simulink model "Regulateur_Proportionel_Integrale"  (R2017a)
settings: Solver=VariableStepAuto  StartTime=0.0  StopTime=20  RelTol=1e-3
values from neighbouring files (symbols this model uses):
  Ti1 = 0.01    [declaration_des_variables.m]
  Ti2 = 0.1    [declaration_des_variables.m]
  Ti3 = 1    [declaration_des_variables.m]
settings Model: Creator=PC  LastModifiedBy=PC

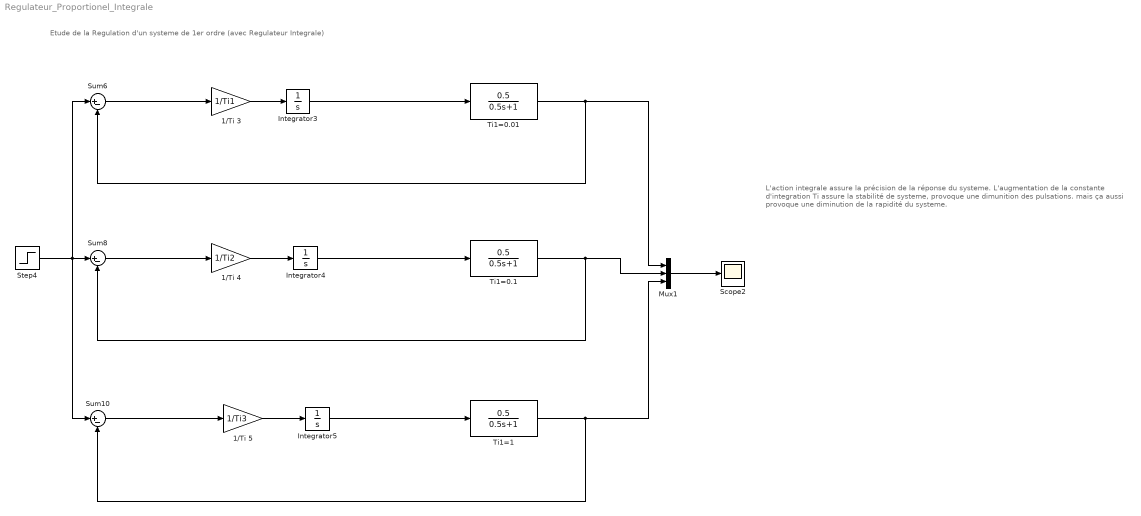
== system Regulateur_Proportionel_Integrale ==
  note: L'action integrale assure la précision de la réponse du systeme.
      | L'augmentation de la constante d'integration Ti assure la stabilité de systeme, provoque une dimunition des pulsations. mais ça aussi provoque une diminution de la rapidité du systeme.
  note: Etude de la Regulation d'un systeme de 1er ordre (avec Regulateur Integrale)
  1/Ti 3 : Gain  Gain=1/Ti1
  1/Ti 4 : Gain  Gain=1/Ti2
  1/Ti 5 : Gain  Gain=1/Ti3
  Integrator3 : Integrator
  Integrator4 : Integrator
  Integrator5 : Integrator
  Mux1 : Mux  Inputs=3
  Scope2 : Scope
  Step4 : Step  Time=0  SampleTime=0
  Sum10 : Sum  Inputs=|+-
  Sum6 : Sum  Inputs=|+-
  Sum8 : Sum  Inputs=|+-
  Ti1=0.01 : TransferFcn  Numerator=[0.5]  Denominator=[0.5 1]
  Ti1=0.1 : TransferFcn  Numerator=[0.5]  Denominator=[0.5 1]
  Ti1=1 : TransferFcn  Numerator=[0.5]  Denominator=[0.5 1]
  wires:
  1/Ti 5/1 -> Integrator5/1
  Integrator5/1 -> Ti1=1/1
  Sum10/1 -> 1/Ti 5/1
  Step4/1 -> Sum10/1, Sum6/1, Sum8/1
  Sum8/1 -> 1/Ti 4/1
  Integrator4/1 -> Ti1=0.1/1
  1/Ti 4/1 -> Integrator4/1
  1/Ti 3/1 -> Integrator3/1
  Integrator3/1 -> Ti1=0.01/1
  Sum6/1 -> 1/Ti 3/1
  Mux1/1 -> Scope2/1
  Ti1=0.1/1 -> Sum8/2, Mux1/2
  Ti1=1/1 -> Mux1/3, Sum10/2
  Ti1=0.01/1 -> Mux1/1, Sum6/2
